simulink model "simplePropagator"  (R2023b)
settings: Solver=VariableStepAuto  StartTime=0.0  StopTime=tf  RelTol=1e-8  AbsTol=1e-8
undefined symbols (not defined in the file): mass, thrust, thrustingThreshold
libraries: vrlib x3, simulink x1
settings Model: Creator=miqui  LastModifiedBy=miqui

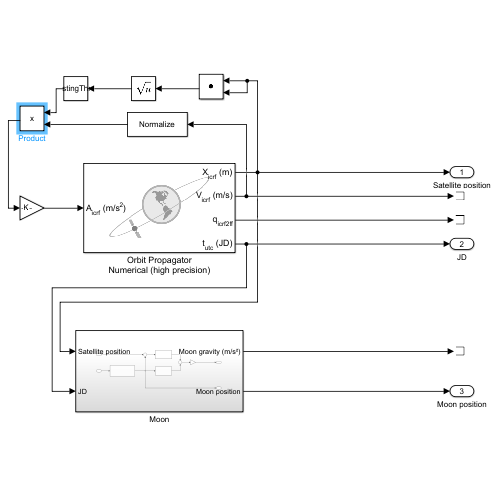
[thumbnail: Simulink's stored preview of the top-level diagram]
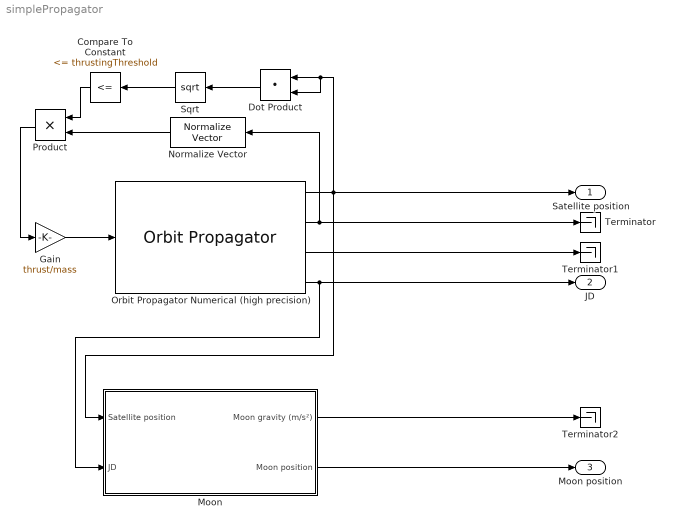
== system simplePropagator ==
  Compare To Constant : simulink/Logic and Bit Operations/Compare To Constant  relop=<=  const=thrustingThreshold  OutDataTypeStr=boolean
  Dot Product : DotProduct  OutDataTypeStr=Inherit: Inherit via internal rule
  Gain : Gain  Gain=thrust/mass
  Moon : Subsystem
  Normalize Vector : vrlib/Utilities/Normalize Vector  maxzero=0
  Orbit Propagator Numerical (high precision) : OrbitPropagator  propagator=Numerical (high precision)  accelIn=on  startDate=startDate  mass=mass  semiMajorAxis=sma  eccentricity=ecc  inclination=inc  raan=RAAN  argPeriapsis=aop  trueAnomaly=true_an  inertialPosition=[3649700.0 3308200.0 -4676600.0]  inertialVelocity=[-2750.8 6666.4 2573.4]  fixedPosition=[-4142689.0 -2676864.7 -4669861.6]  fixedVelocity=[1452.7 -6720.7 2568.1]  gravityModel=Point-mass  customR=3396200  customMu=4.305e13  customJ2=1.0826269e-03  customOmega=4.06125949e-3  useEOPs=off  outputTransform=on  useThirdBodyGravity=on  includeSunGravity=off  useSRP=on  srpArea=area
  Product : Product
  Sqrt : Sqrt
  Terminator : Terminator
  Terminator1 : Terminator
  Terminator2 : Terminator
  Satellite position : Outport
  JD : Outport  Port=2
  Moon position : Outport  Port=3
  wires:
  Orbit Propagator Numerical (high precision)/2 -> Normalize Vector/1, Terminator/1
  Orbit Propagator Numerical (high precision)/3 -> Terminator1/1
  Orbit Propagator Numerical (high precision)/4 -> Moon/2(JD), JD/1
  Moon/2(Moon position) -> Moon position/1
  Moon/1(Moon gravity (m/s²)) -> Terminator2/1
  Gain/1 -> Orbit Propagator Numerical (high precision)/1
  Compare To Constant/1 -> Product/1
  Normalize Vector/1 -> Product/2
  Product/1 -> Gain/1
  Orbit Propagator Numerical (high precision)/1 -> Dot Product/2, Dot Product/1, Moon/1(Satellite position), Satellite position/1
  Dot Product/1 -> Sqrt/1
  Sqrt/1 -> Compare To Constant/1

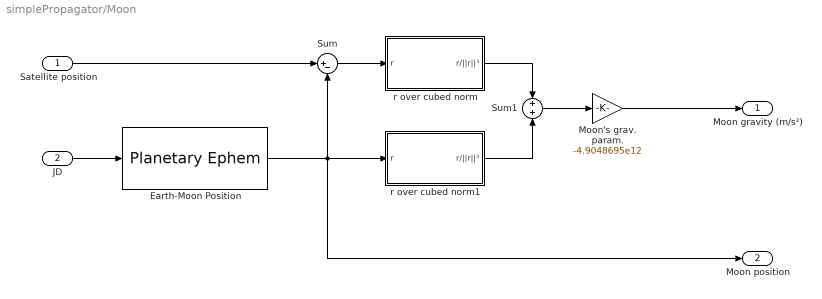
== system simplePropagator/Moon ==
  Satellite position : Inport
  JD : Inport  Port=2
  Earth-Moon Position : PlanetaryEphem  units=m,m/s  useDateRange=on  outputVelocity=off
  Moon's grav. param. : Gain  Gain=-4.9048695e12
  Sum : Sum  Inputs=|+-
  Sum1 : Sum
  r over cubed norm : Subsystem
  r over cubed norm1 : Subsystem
  Moon gravity (m/s²) : Outport
  Moon position : Outport  Port=2
  wires:
  JD/1 -> Earth-Moon Position/1
  Satellite position/1 -> Sum/1
  Earth-Moon Position/1 -> Moon position/1, r over cubed norm1/1(r), Sum/2
  Sum/1 -> r over cubed norm/1(r)
  Sum1/1 -> Moon's grav. param./1
  Moon's grav. param./1 -> Moon gravity (m/s²)/1
  r over cubed norm/1(r/||r||³) -> Sum1/1
  r over cubed norm1/1(r/||r||³) -> Sum1/2

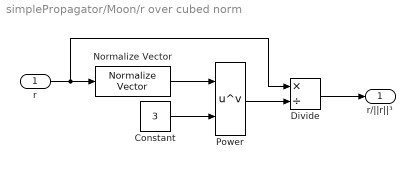
== system simplePropagator/Moon/r over cubed norm ==
  r : Inport
  Constant : Constant  Value=3
  Divide : Product  Inputs=*/
  Normalize Vector : vrlib/Utilities/Normalize Vector  maxzero=0
  Power : Math  Operator=pow
  r/||r||³ : Outport
  wires:
  r/1 -> Divide/1, Normalize Vector/1
  Normalize Vector/1 -> Power/1
  Constant/1 -> Power/2
  Power/1 -> Divide/2
  Divide/1 -> r/||r||³/1

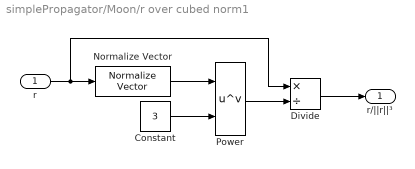
== system simplePropagator/Moon/r over cubed norm1 ==
  r : Inport
  Constant : Constant  Value=3
  Divide : Product  Inputs=*/
  Normalize Vector : vrlib/Utilities/Normalize Vector  maxzero=0
  Power : Math  Operator=pow
  r/||r||³ : Outport
  wires:
  r/1 -> Divide/1, Normalize Vector/1
  Normalize Vector/1 -> Power/1
  Constant/1 -> Power/2
  Power/1 -> Divide/2
  Divide/1 -> r/||r||³/1
